simulink subsystem "PC_SS"  (R2022a)
settings: Solver=VariableStepAuto  StartTime=0.0  StopTime=10.0  RelTol=1e-3
libraries: hdlBasic x5
settings Model: Creator=viktor  LastModifiedBy=viktor

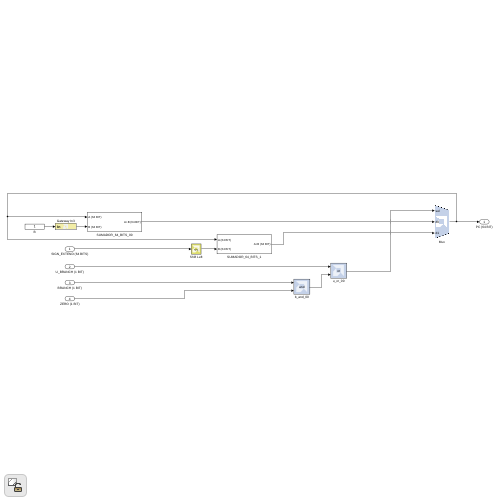
[thumbnail: Simulink's stored preview of the top-level diagram]
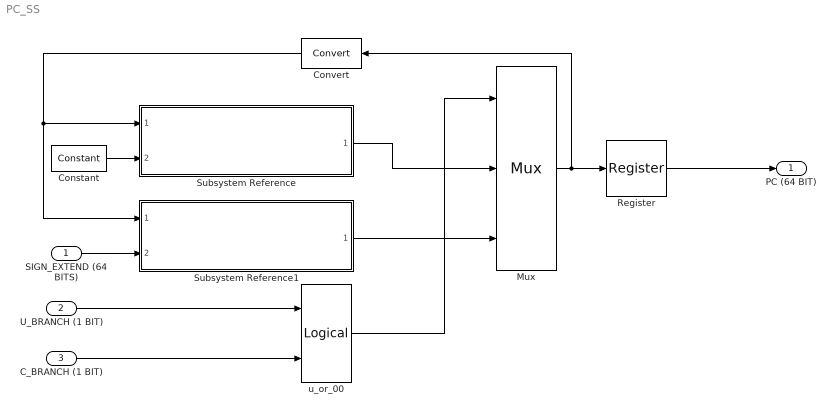
== system PC_SS ==
  SIGN_EXTEND (64 BITS) : Inport
  U_BRANCH (1 BIT) : Inport  Port=2
  C_BRANCH (1 BIT) : Inport  Port=3
  Constant : hdlBasic/Constant  const=1.0  gui_display_data_type=Fixed-point  arith_type=Unsigned  n_bits=64  bin_pt=0  preci_type=Single  exp_width=8  frac_width=24  explicit_period=off  period=1  XmcBlockStatus=1  maskContainerNames=tabcontainer1  block_type=constant  block_config=sysgen:Constant_config
  Convert : hdlBasic/Convert  gui_display_data_type=Fixed-point  arith_type=Unsigned  n_bits=64  bin_pt=0  float_type=Single  exp_bits=8  fraction_bits=24  quantization=Truncate  overflow=Wrap  en=off  latency=1  pipeline=off  XmcBlockStatus=1  maskContainerNames=group2  block_type=convert  block_config=sysgen:Convert_config  block_width=595  block_height=885
  Mux : hdlBasic/Mux  inputs=2  en=off  latency=0  precision=Full  arith_type=Unsigned  n_bits=16  bin_pt=14  quantization=Truncate  overflow=Wrap  XmcBlockStatus=1  maskContainerNames=tabcontainer1  block_type=mux  block_config=sysgen:Mux_config
  Register : hdlBasic/Register  init=0  rst=off  en=off  XmcBlockStatus=1  maskContainerNames=tabcontainer1  block_type=register  block_config=sysgen:Register_config
  Subsystem Reference : Subsystem  ReferencedSubsystem=SUMADOR_64_BITS_SS
  Subsystem Reference1 : Subsystem  ReferencedSubsystem=SUMADOR_64_BITS_SS
  u_or_00 : hdlBasic/Logical  logical_function=OR  inputs=2  en=off  latency=0  precision=User Defined  arith_type=Boolean  n_bits=16  bin_pt=0  align_bp=on  overflow=[]  quantization=[]  XmcBlockStatus=1  maskContainerNames=tabcontainer1  block_type=logical  block_config=sysgen:Logical_config
  PC (64 BIT) : Outport
  wires:
  Subsystem Reference1/1 -> Mux/3
  Subsystem Reference/1 -> Mux/2
  u_or_00/1 -> Mux/1
  Mux/1 -> Register/1, Convert/1
  C_BRANCH (1 BIT)/1 -> u_or_00/2
  Register/1 -> PC (64 BIT)/1
  Convert/1 -> Subsystem Reference1/1, Subsystem Reference/1
  Constant/1 -> Subsystem Reference/2
  U_BRANCH (1 BIT)/1 -> u_or_00/1
  SIGN_EXTEND (64 BITS)/1 -> Subsystem Reference1/2
